simulink model "case2"  (R2024b)
settings: Solver=FixedStepAuto  StartTime=0  StopTime=1  FixedStep=1e-7  RelTol=1e-3
values from neighbouring files (symbols this model uses):
  SG_D_1_D = 0.01056    [IEEE9_case_parameters.m]    (also in case1_parameters.m; case2_parameters.m; case3_parameters.m; case4_parameters.m)
  SG_D_1_EnableSaturation = 0    [IEEE9_case_parameters.m]    (also in case1_parameters.m; case2_parameters.m; case3_parameters.m; case4_parameters.m)
  SG_D_1_f0 = 60    [IEEE9_case_parameters.m]    (also in case1_parameters.m; case2_parameters.m; case3_parameters.m; case4_parameters.m)
  SG_D_1_H = 7.5    [IEEE9_case_parameters.m]    (also in case1_parameters.m; case2_parameters.m; case3_parameters.m; case4_parameters.m)
  SG_D_1_K_A = 20    [IEEE9_case_parameters.m]    (also in case1_parameters.m; case2_parameters.m; case3_parameters.m; case4_parameters.m)
  SG_D_1_K_E = 1.000000e+1    (= 10)    [IEEE9_case_parameters.m]    (also in case1_parameters.m; case2_parameters.m; case3_parameters.m; case4_parameters.m)
  SG_D_1_K_F = 2.363    [IEEE9_case_parameters.m]    (also in case1_parameters.m; case2_parameters.m; case3_parameters.m; case4_parameters.m)
  SG_D_1_K_s = 0.5    [IEEE9_case_parameters.m]    (also in case1_parameters.m = 5; case2_parameters.m = 5; case3_parameters.m = 5; case4_parameters.m = 5)
  SG_D_1_R_a = 0.001088    [IEEE9_case_parameters.m]    (also in case1_parameters.m; case2_parameters.m; case3_parameters.m; case4_parameters.m)
  SG_D_1_S_A = 1    [IEEE9_case_parameters.m]    (also in case1_parameters.m; case2_parameters.m; case3_parameters.m; case4_parameters.m)
  SG_D_1_S_B = 0.103    [IEEE9_case_parameters.m]    (also in case1_parameters.m; case2_parameters.m; case3_parameters.m; case4_parameters.m)
  SG_D_1_S_N = 10.659857    [IEEE9_case_parameters.m]    (also in case1_parameters.m; case2_parameters.m; case3_parameters.m; case4_parameters.m)
  SG_D_1_SpeedPara = 200    [IEEE9_case_parameters.m]    (also in case1_parameters.m; case2_parameters.m; case3_parameters.m; case4_parameters.m)
  SG_D_1_T_0 = 0.720173    [IEEE9_case_parameters.m]    (also in case1_parameters.m = 0.755522; case2_parameters.m = 0.808931; case3_parameters.m = 0.869402; case4_parameters.m = 0.729316)
  SG_D_1_T_1 = 0.3    [IEEE9_case_parameters.m]    (also in case1_parameters.m; case2_parameters.m; case3_parameters.m; case4_parameters.m)
  SG_D_1_T_2 = 0.05    [IEEE9_case_parameters.m]    (also in case1_parameters.m; case2_parameters.m; case3_parameters.m; case4_parameters.m)
  SG_D_1_T_3 = 0.02    [IEEE9_case_parameters.m]    (also in case1_parameters.m; case2_parameters.m; case3_parameters.m; case4_parameters.m)
  SG_D_1_T_4 = 0.005    [IEEE9_case_parameters.m]    (also in case1_parameters.m; case2_parameters.m; case3_parameters.m; case4_parameters.m)
  SG_D_1_T_A = 0.02    [IEEE9_case_parameters.m]    (also in case1_parameters.m; case2_parameters.m; case3_parameters.m; case4_parameters.m)
  SG_D_1_T_dd = 8.000000e+0    (= 8)    [IEEE9_case_parameters.m]    (also in case1_parameters.m; case2_parameters.m; case3_parameters.m; case4_parameters.m)
  SG_D_1_T_ddd = 0.04    [IEEE9_case_parameters.m]    (also in case1_parameters.m; case2_parameters.m; case3_parameters.m; case4_parameters.m)
  SG_D_1_T_E = 0.314    [IEEE9_case_parameters.m]    (also in case1_parameters.m; case2_parameters.m; case3_parameters.m; case4_parameters.m)
  SG_D_1_T_F = 0.35    [IEEE9_case_parameters.m]    (also in case1_parameters.m; case2_parameters.m; case3_parameters.m; case4_parameters.m)
  SG_D_1_T_qd = 0.8    [IEEE9_case_parameters.m]    (also in case1_parameters.m; case2_parameters.m; case3_parameters.m; case4_parameters.m)
  SG_D_1_T_qdd = 0.02    [IEEE9_case_parameters.m]    (also in case1_parameters.m; case2_parameters.m; case3_parameters.m; case4_parameters.m)
  SG_D_1_T_speed = 0.1    [IEEE9_case_parameters.m]    (also in case1_parameters.m = 200; case2_parameters.m = 200; case3_parameters.m = 200; case4_parameters.m = 200)
  SG_D_1_T_w = 0.5    [IEEE9_case_parameters.m]    (also in case1_parameters.m; case2_parameters.m; case3_parameters.m; case4_parameters.m)
  SG_D_1_V_ref = 1.990276    [IEEE9_case_parameters.m]    (also in case1_parameters.m = 2.042296; case2_parameters.m = 2.051388; case3_parameters.m = 2.089584; case4_parameters.m = 2.01845)
  SG_D_1_w_ref = 376.991118    [IEEE9_case_parameters.m]    (also in case1_parameters.m; case2_parameters.m; case3_parameters.m; case4_parameters.m)
  SG_D_1_wb = 6.000000e+1    (= 60)    [IEEE9_case_parameters.m]    (also in case1_parameters.m; case2_parameters.m; case3_parameters.m; case4_parameters.m)
  SG_D_1_x_d = 1.9    [IEEE9_case_parameters.m]    (also in case1_parameters.m; case2_parameters.m; case3_parameters.m; case4_parameters.m)
  SG_D_1_x_dd = 0.302    [IEEE9_case_parameters.m]    (also in case1_parameters.m; case2_parameters.m; case3_parameters.m; case4_parameters.m)
  SG_D_1_x_ddd = 0.204    [IEEE9_case_parameters.m]    (also in case1_parameters.m; case2_parameters.m; case3_parameters.m; case4_parameters.m)
  SG_D_1_x_l = 0.05    [IEEE9_case_parameters.m]    (also in case1_parameters.m; case2_parameters.m; case3_parameters.m; case4_parameters.m)
  SG_D_1_x_q = 1.3    [IEEE9_case_parameters.m]    (also in case1_parameters.m; case2_parameters.m; case3_parameters.m; case4_parameters.m)
  SG_D_1_x_qd = 0.5    [IEEE9_case_parameters.m]    (also in case1_parameters.m; case2_parameters.m; case3_parameters.m; case4_parameters.m)
  SG_D_1_x_qdd = 0.3    [IEEE9_case_parameters.m]    (also in case1_parameters.m; case2_parameters.m; case3_parameters.m; case4_parameters.m)
  SG_D_2_D = 0.02    [IEEE9_case_parameters.m]    (also in case1_parameters.m; case2_parameters.m; case3_parameters.m; case4_parameters.m)
  SG_D_2_EnableSaturation = 0    [IEEE9_case_parameters.m]    (also in case1_parameters.m; case2_parameters.m; case3_parameters.m; case4_parameters.m)
  SG_D_2_f0 = 60    [IEEE9_case_parameters.m]    (also in case1_parameters.m; case2_parameters.m; case3_parameters.m; case4_parameters.m)
  SG_D_2_H = 8.000000e+0    (= 8)    [IEEE9_case_parameters.m]    (also in case1_parameters.m; case2_parameters.m; case3_parameters.m; case4_parameters.m)
  SG_D_2_K_A = 20    [IEEE9_case_parameters.m]    (also in case1_parameters.m; case2_parameters.m; case3_parameters.m; case4_parameters.m)
  SG_D_2_K_E = 1.000000e+1    (= 10)    [IEEE9_case_parameters.m]    (also in case1_parameters.m; case2_parameters.m; case3_parameters.m; case4_parameters.m)
  SG_D_2_K_F = 2.363    [IEEE9_case_parameters.m]    (also in case1_parameters.m; case2_parameters.m; case3_parameters.m; case4_parameters.m)
  SG_D_2_K_s = 0.5    [IEEE9_case_parameters.m]    (also in case1_parameters.m = 4; case2_parameters.m = 4; case3_parameters.m = 4; case4_parameters.m = 4)
  SG_D_2_R_a = 0.001088    [IEEE9_case_parameters.m]    (also in case1_parameters.m; case2_parameters.m; case3_parameters.m; case4_parameters.m)
  SG_D_2_S_A = 1    [IEEE9_case_parameters.m]    (also in case1_parameters.m; case2_parameters.m; case3_parameters.m; case4_parameters.m)
  SG_D_2_S_B = 0.103    [IEEE9_case_parameters.m]    (also in case1_parameters.m; case2_parameters.m; case3_parameters.m; case4_parameters.m)
  SG_D_2_S_N = 10.659857    [IEEE9_case_parameters.m]    (also in case1_parameters.m; case2_parameters.m; case3_parameters.m; case4_parameters.m)
  SG_D_2_SpeedPara = 200    [IEEE9_case_parameters.m]    (also in case1_parameters.m; case2_parameters.m; case3_parameters.m; case4_parameters.m)
  SG_D_2_T_0 = 1.632913    [IEEE9_case_parameters.m]    (also in case1_parameters.m = 1.632925; case2_parameters.m = 1.632915; case3_parameters.m = 1.632914; case4_parameters.m = 1.632927)
  SG_D_2_T_1 = 0.2    [IEEE9_case_parameters.m]    (also in case1_parameters.m; case2_parameters.m; case3_parameters.m; case4_parameters.m)
  SG_D_2_T_2 = 0.05    [IEEE9_case_parameters.m]    (also in case1_parameters.m; case2_parameters.m; case3_parameters.m; case4_parameters.m)
  SG_D_2_T_3 = 0.02    [IEEE9_case_parameters.m]    (also in case1_parameters.m; case2_parameters.m; case3_parameters.m; case4_parameters.m)
  SG_D_2_T_4 = 0.005    [IEEE9_case_parameters.m]    (also in case1_parameters.m; case2_parameters.m; case3_parameters.m; case4_parameters.m)
  SG_D_2_T_A = 0.02    [IEEE9_case_parameters.m]    (also in case1_parameters.m; case2_parameters.m; case3_parameters.m; case4_parameters.m)
  SG_D_2_T_dd = 7.9    [IEEE9_case_parameters.m]    (also in case1_parameters.m; case2_parameters.m; case3_parameters.m; case4_parameters.m)
  SG_D_2_T_ddd = 0.04    [IEEE9_case_parameters.m]    (also in case1_parameters.m; case2_parameters.m; case3_parameters.m; case4_parameters.m)
  SG_D_2_T_E = 0.314    [IEEE9_case_parameters.m]    (also in case1_parameters.m; case2_parameters.m; case3_parameters.m; case4_parameters.m)
  SG_D_2_T_F = 0.35    [IEEE9_case_parameters.m]    (also in case1_parameters.m; case2_parameters.m; case3_parameters.m; case4_parameters.m)
  SG_D_2_T_qd = 0.8    [IEEE9_case_parameters.m]    (also in case1_parameters.m; case2_parameters.m; case3_parameters.m; case4_parameters.m)
  SG_D_2_T_qdd = 0.015    [IEEE9_case_parameters.m]    (also in case1_parameters.m; case2_parameters.m; case3_parameters.m; case4_parameters.m)
  SG_D_2_T_speed = 0.1    [IEEE9_case_parameters.m]    (also in case1_parameters.m = 150; case2_parameters.m = 150; case3_parameters.m = 150; case4_parameters.m = 150)
  SG_D_2_T_w = 0.35    [IEEE9_case_parameters.m]    (also in case1_parameters.m; case2_parameters.m; case3_parameters.m; case4_parameters.m)
  SG_D_2_V_ref = 2.58547    [IEEE9_case_parameters.m]    (also in case1_parameters.m = 2.597896; case2_parameters.m = 2.587136; case3_parameters.m = 2.586042; case4_parameters.m = 2.599679)
  SG_D_2_w_ref = 376.991118    [IEEE9_case_parameters.m]    (also in case1_parameters.m; case2_parameters.m; case3_parameters.m; case4_parameters.m)
  SG_D_2_wb = 6.000000e+1    (= 60)    [IEEE9_case_parameters.m]    (also in case1_parameters.m; case2_parameters.m; case3_parameters.m; case4_parameters.m)
  SG_D_2_x_d = 1.8    [IEEE9_case_parameters.m]    (also in case1_parameters.m; case2_parameters.m; case3_parameters.m; case4_parameters.m)
  SG_D_2_x_dd = 0.302    [IEEE9_case_parameters.m]    (also in case1_parameters.m; case2_parameters.m; case3_parameters.m; case4_parameters.m)
  SG_D_2_x_ddd = 0.204    [IEEE9_case_parameters.m]    (also in case1_parameters.m; case2_parameters.m; case3_parameters.m; case4_parameters.m)
  SG_D_2_x_l = 0.05    [IEEE9_case_parameters.m]    (also in case1_parameters.m; case2_parameters.m; case3_parameters.m; case4_parameters.m)
  SG_D_2_x_q = 1.25    [IEEE9_case_parameters.m]    (also in case1_parameters.m; case2_parameters.m; case3_parameters.m; case4_parameters.m)
  SG_D_2_x_qd = 0.5    [IEEE9_case_parameters.m]    (also in case1_parameters.m; case2_parameters.m; case3_parameters.m; case4_parameters.m)
  SG_D_2_x_qdd = 0.3    [IEEE9_case_parameters.m]    (also in case1_parameters.m; case2_parameters.m; case3_parameters.m; case4_parameters.m)
  SG_D_3_D = 0.02    [IEEE9_case_parameters.m]    (also in case1_parameters.m; case2_parameters.m; case3_parameters.m; case4_parameters.m)
  SG_D_3_EnableSaturation = 0    [IEEE9_case_parameters.m]    (also in case1_parameters.m; case2_parameters.m; case3_parameters.m; case4_parameters.m)
  SG_D_3_f0 = 60    [IEEE9_case_parameters.m]    (also in case1_parameters.m; case2_parameters.m; case3_parameters.m; case4_parameters.m)
  SG_D_3_H = 7.7    [IEEE9_case_parameters.m]    (also in case1_parameters.m; case2_parameters.m; case3_parameters.m; case4_parameters.m)
  SG_D_3_K_A = 20    [IEEE9_case_parameters.m]    (also in case1_parameters.m; case2_parameters.m; case3_parameters.m; case4_parameters.m)
  SG_D_3_K_E = 1.000000e+1    (= 10)    [IEEE9_case_parameters.m]    (also in case1_parameters.m; case2_parameters.m; case3_parameters.m; case4_parameters.m)
  SG_D_3_K_F = 2.363    [IEEE9_case_parameters.m]    (also in case1_parameters.m; case2_parameters.m; case3_parameters.m; case4_parameters.m)
  SG_D_3_K_s = 0.2    [IEEE9_case_parameters.m]    (also in case1_parameters.m = 2; case2_parameters.m = 2; case3_parameters.m = 2; case4_parameters.m = 2)
  SG_D_3_R_a = 0.001088    [IEEE9_case_parameters.m]    (also in case1_parameters.m; case2_parameters.m; case3_parameters.m; case4_parameters.m)
  SG_D_3_S_A = 1    [IEEE9_case_parameters.m]    (also in case1_parameters.m; case2_parameters.m; case3_parameters.m; case4_parameters.m)
  SG_D_3_S_B = 0.103    [IEEE9_case_parameters.m]    (also in case1_parameters.m; case2_parameters.m; case3_parameters.m; case4_parameters.m)
  SG_D_3_S_N = 10.659857    [IEEE9_case_parameters.m]    (also in case1_parameters.m; case2_parameters.m; case3_parameters.m; case4_parameters.m)
  SG_D_3_SpeedPara = 200    [IEEE9_case_parameters.m]    (also in case1_parameters.m; case2_parameters.m; case3_parameters.m; case4_parameters.m)
  SG_D_3_T_0 = 0.850788    [IEEE9_case_parameters.m]    (also in case1_parameters.m = 0.850786; case2_parameters.m = 0.850787; case3_parameters.m; case4_parameters.m = 0.850786)
  SG_D_3_T_1 = 0.2    [IEEE9_case_parameters.m]    (also in case1_parameters.m; case2_parameters.m; case3_parameters.m; case4_parameters.m)
  SG_D_3_T_2 = 0.05    [IEEE9_case_parameters.m]    (also in case1_parameters.m; case2_parameters.m; case3_parameters.m; case4_parameters.m)
  SG_D_3_T_3 = 0.02    [IEEE9_case_parameters.m]    (also in case1_parameters.m; case2_parameters.m; case3_parameters.m; case4_parameters.m)
  SG_D_3_T_4 = 0.005    [IEEE9_case_parameters.m]    (also in case1_parameters.m; case2_parameters.m; case3_parameters.m; case4_parameters.m)
  SG_D_3_T_A = 0.02    [IEEE9_case_parameters.m]    (also in case1_parameters.m; case2_parameters.m; case3_parameters.m; case4_parameters.m)
  SG_D_3_T_dd = 8.1    [IEEE9_case_parameters.m]    (also in case1_parameters.m; case2_parameters.m; case3_parameters.m; case4_parameters.m)
  SG_D_3_T_ddd = 0.04    [IEEE9_case_parameters.m]    (also in case1_parameters.m; case2_parameters.m; case3_parameters.m; case4_parameters.m)
  SG_D_3_T_E = 0.314    [IEEE9_case_parameters.m]    (also in case1_parameters.m; case2_parameters.m; case3_parameters.m; case4_parameters.m)
  SG_D_3_T_F = 0.35    [IEEE9_case_parameters.m]    (also in case1_parameters.m; case2_parameters.m; case3_parameters.m; case4_parameters.m)
  SG_D_3_T_qd = 0.8    [IEEE9_case_parameters.m]    (also in case1_parameters.m; case2_parameters.m; case3_parameters.m; case4_parameters.m)
  SG_D_3_T_qdd = 0.015    [IEEE9_case_parameters.m]    (also in case1_parameters.m; case2_parameters.m; case3_parameters.m; case4_parameters.m)
  SG_D_3_T_speed = 0.1    [IEEE9_case_parameters.m]    (also in case1_parameters.m = 180; case2_parameters.m = 180; case3_parameters.m = 180; case4_parameters.m = 180)
  SG_D_3_T_w = 0.4    [IEEE9_case_parameters.m]    (also in case1_parameters.m; case2_parameters.m; case3_parameters.m; case4_parameters.m)
  SG_D_3_V_ref = 1.892727    [IEEE9_case_parameters.m]    (also in case1_parameters.m = 1.906439; case2_parameters.m = 1.895535; case3_parameters.m = 1.892105; case4_parameters.m = 1.906598)
  SG_D_3_w_ref = 376.991118    [IEEE9_case_parameters.m]    (also in case1_parameters.m; case2_parameters.m; case3_parameters.m; case4_parameters.m)
  SG_D_3_wb = 6.000000e+1    (= 60)    [IEEE9_case_parameters.m]    (also in case1_parameters.m; case2_parameters.m; case3_parameters.m; case4_parameters.m)
  SG_D_3_x_d = 1.85    [IEEE9_case_parameters.m]    (also in case1_parameters.m; case2_parameters.m; case3_parameters.m; case4_parameters.m)
  SG_D_3_x_dd = 0.302    [IEEE9_case_parameters.m]    (also in case1_parameters.m; case2_parameters.m; case3_parameters.m; case4_parameters.m)
  SG_D_3_x_ddd = 0.204    [IEEE9_case_parameters.m]    (also in case1_parameters.m; case2_parameters.m; case3_parameters.m; case4_parameters.m)
  SG_D_3_x_l = 0.05    [IEEE9_case_parameters.m]    (also in case1_parameters.m; case2_parameters.m; case3_parameters.m; case4_parameters.m)
  SG_D_3_x_q = 1.2    [IEEE9_case_parameters.m]    (also in case1_parameters.m; case2_parameters.m; case3_parameters.m; case4_parameters.m)
  SG_D_3_x_qd = 0.5    [IEEE9_case_parameters.m]    (also in case1_parameters.m; case2_parameters.m; case3_parameters.m; case4_parameters.m)
  SG_D_3_x_qdd = 0.3    [IEEE9_case_parameters.m]    (also in case1_parameters.m; case2_parameters.m; case3_parameters.m; case4_parameters.m)
(part 9 of 12)

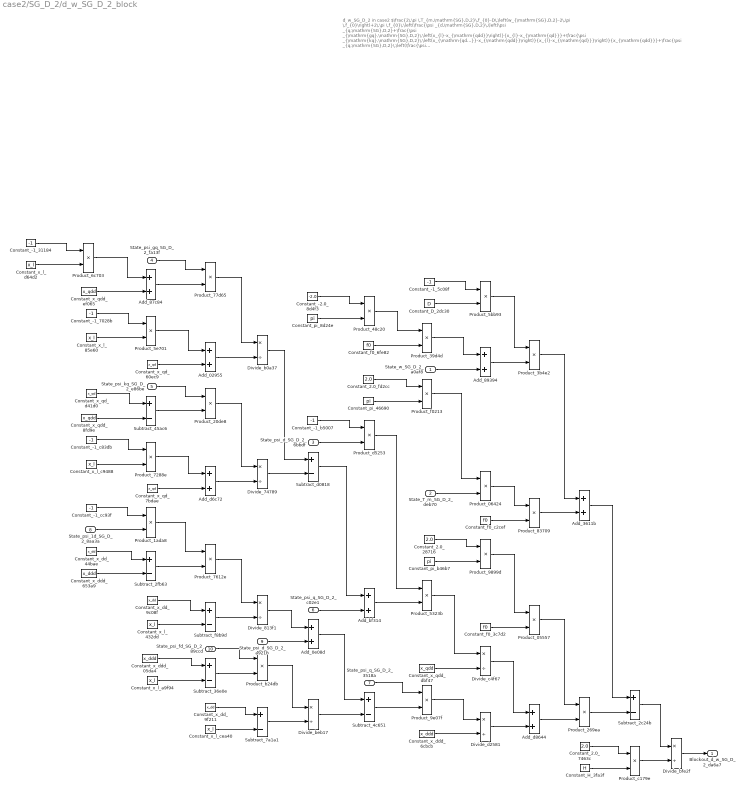
== system case2/SG_D_2/d_w_SG_D_2_block ==
  note: d_w_SG_D_2 in case2
      | $\frac{2\,\pi \,T_{m,\mathrm{SG},D,2}\,f_{0}-D\,\left(w_{\mathrm{SG},D,2}-2\,\pi \,f_{0}\right)+2\,\pi \,f_{0}\,\left(\frac{\psi _{d,\mathrm{SG},D,2}\,\left(\psi _{q,\mathrm{SG},D,2}+\frac{\psi _{\mathrm{gq},\mathrm{SG},D,2}\,\left(x_{l}-x_{\mathrm{qdd}}\right)}{x_{l}-x_{\mathrm{qd}}}+\frac{\psi _{\mathrm{kq},\mathrm{SG},D,2}\,\left(x_{\mathrm{qd}}-x_{\mathrm{qdd}}\right)}{x_{l}-x_{\mathrm{qd}}}\right)}{x_{\mathrm{qdd}}}+\frac{\psi _{q,\mathrm{SG},D,2}\,\left(\frac{\psi _{\mathrm{1d},\mathrm{SG},D,2}\,\left(x_{\mathrm{dd}}-x_{\mathrm{ddd}}\right)}{x_{\mathrm{dd}}-x_{l}}-\psi _{d,\mathrm{SG},D,2}+\frac{\psi _{\mathrm{fd},\mathrm{SG},D,2}\,\left(x_{\mathrm{ddd}}-x_{l}\right)}{x_{\mathrm{dd}}-x_{l}}\right)}{x_{\mathrm{ddd}}}\right)}{2\,H}$
      | Automatically generated on 2025-10-31 18:54:39 .
  State_w_SG_D_2_a0af8 : Inport
  State_T_m_SG_D_2_deb70 : Inport  Port=2
  State_psi_d_SG_D_2_6bbdf : Inport  Port=3
  State_psi_gq_SG_D_2_fa13f : Inport  Port=4
  State_psi_kq_SG_D_2_e86be : Inport  Port=5
  State_psi_q_SG_D_2_c02e1 : Inport  Port=6
  State_psi_q_SG_D_2_3518a : Inport  Port=7
  State_psi_1d_SG_D_2_8aa3a : Inport  Port=8
  State_psi_d_SG_D_2_a921b : Inport  Port=9
  State_psi_fd_SG_D_2_89ccd : Inport  Port=10
  Add_02955 : Sum
  Add_0e08d : Sum
  Add_3611b : Sum
  Add_87c84 : Sum
  Add_89394 : Sum
  Add_bf314 : Sum
  Add_d6c72 : Sum
  Add_d8644 : Sum
  Constant_-1_31184 : Constant  Value=-1
  Constant_-1_5c08f : Constant  Value=-1
  Constant_-1_7028b : Constant  Value=-1
  Constant_-1_b5007 : Constant  Value=-1
  Constant_-1_c83db : Constant  Value=-1
  Constant_-1_cc93f : Constant  Value=-1
  Constant_-2.0_8d4f3 : Constant  Value=-2.0
  Constant_2.0_28716 : Constant  Value=2.0
  Constant_2.0_7463c : Constant  Value=2.0
  Constant_2.0_fd2cc : Constant  Value=2.0
  Constant_D_2dc30 : Constant  Value=D
  Constant_H_3fa3f : Constant  Value=H
  Constant_f0_3c7d2 : Constant  Value=f0
  Constant_f0_6fe82 : Constant  Value=f0
  Constant_f0_c2cef : Constant  Value=f0
  Constant_pi_46690 : Constant  Value=pi
  Constant_pi_8d24e : Constant  Value=pi
  Constant_pi_b46b7 : Constant  Value=pi
  Constant_x_dd_44bae : Constant  Value=x_dd
  Constant_x_dd_9c08f : Constant  Value=x_dd
  Constant_x_dd_9f211 : Constant  Value=x_dd
  Constant_x_ddd_05da4 : Constant  Value=x_ddd
  Constant_x_ddd_653a9 : Constant  Value=x_ddd
  Constant_x_ddd_6cbcb : Constant  Value=x_ddd
  Constant_x_l_432dd : Constant  Value=x_l
  Constant_x_l_85e60 : Constant  Value=x_l
  Constant_x_l_a9f94 : Constant  Value=x_l
  Constant_x_l_c9488 : Constant  Value=x_l
  Constant_x_l_cea40 : Constant  Value=x_l
  Constant_x_l_d64d2 : Constant  Value=x_l
  Constant_x_qd_60ec9 : Constant  Value=x_qd
  Constant_x_qd_7bdae : Constant  Value=x_qd
  Constant_x_qd_d41d0 : Constant  Value=x_qd
  Constant_x_qdd_8fd9e : Constant  Value=x_qdd
  Constant_x_qdd_dbf47 : Constant  Value=x_qdd
  Constant_x_qdd_ef065 : Constant  Value=x_qdd
  Divide_74789 : Product  Inputs=*/
  Divide_813f1 : Product  Inputs=*/
  Divide_b0a37 : Product  Inputs=*/
  Divide_beb17 : Product  Inputs=*/
  Divide_bfe2f : Product  Inputs=*/
  Divide_c4f67 : Product  Inputs=*/
  Divide_d2581 : Product  Inputs=*/
  Product_05557 : Product
  Product_06424 : Product
  Product_1ada8 : Product
  Product_20de8 : Product
  Product_269ea : Product
  Product_39d4d : Product
  Product_3b4e2 : Product
  Product_48c20 : Product
  Product_5323b : Product
  Product_5bb93 : Product
  Product_5e701 : Product
  Product_6c703 : Product
  Product_7288e : Product
  Product_7612e : Product
  Product_77d65 : Product
  Product_83709 : Product
  Product_9899d : Product
  Product_9e07f : Product
  Product_b24db : Product
  Product_c179e : Product
  Product_d5253 : Product
  Product_f0213 : Product
  Subtract_2c24b : Sum  Inputs=+-
  Subtract_2fb63 : Sum  Inputs=+-
  Subtract_36e0e : Sum  Inputs=+-
  Subtract_45ac6 : Sum  Inputs=+-
  Subtract_4c651 : Sum  Inputs=+-
  Subtract_7a1a1 : Sum  Inputs=+-
  Subtract_d0818 : Sum  Inputs=+-
  Subtract_f8b9d : Sum  Inputs=+-
  Blockout_d_w_SG_D_2_da6a7 : Outport
  wires:
  Constant_x_qd_d41d0/1 -> Subtract_45ac6/1
  Constant_-1_c83db/1 -> Product_7288e/1
  Constant_-1_31184/1 -> Product_6c703/1
  Constant_x_qdd_8fd9e/1 -> Subtract_45ac6/2
  Subtract_7a1a1/1 -> Divide_beb17/2
  Constant_x_l_c9488/1 -> Product_7288e/2
  Constant_x_l_d64d2/1 -> Product_6c703/2
  Product_7288e/1 -> Add_d6c72/1
  Product_6c703/1 -> Add_87c84/1
  Constant_x_l_432dd/1 -> Subtract_f8b9d/2
  Constant_x_l_85e60/1 -> Product_5e701/2
  Constant_x_ddd_6cbcb/1 -> Divide_d2581/2
  Subtract_36e0e/1 -> Product_b24db/2
  Constant_x_qd_7bdae/1 -> Add_d6c72/2
  Constant_x_qdd_ef065/1 -> Add_87c84/2
  Constant_-1_7028b/1 -> Product_5e701/1
  State_psi_d_SG_D_2_6bbdf/1 -> Product_d5253/2
  Constant_-1_cc93f/1 -> Product_1ada8/1
  State_w_SG_D_2_a0af8/1 -> Add_89394/2
  Product_5e701/1 -> Add_02955/1
  State_psi_1d_SG_D_2_8aa3a/1 -> Product_1ada8/2
  Constant_x_dd_44bae/1 -> Subtract_2fb63/1
  Divide_b0a37/1 -> Subtract_d0818/1
  Subtract_45ac6/1 -> Product_20de8/2
  Constant_x_ddd_653a9/1 -> Subtract_2fb63/2
  State_psi_gq_SG_D_2_fa13f/1 -> Product_77d65/1
  Add_d6c72/1 -> Divide_74789/2
  State_psi_d_SG_D_2_a921b/1 -> Add_0e08d/2
  Add_87c84/1 -> Product_77d65/2
  Constant_x_qd_60ec9/1 -> Add_02955/2
  State_psi_kq_SG_D_2_e86be/1 -> Product_20de8/1
  Product_1ada8/1 -> Product_7612e/1
  Subtract_2fb63/1 -> Product_7612e/2
  Constant_pi_46690/1 -> Product_f0213/2
  Constant_x_dd_9c08f/1 -> Subtract_f8b9d/1
  Constant_x_ddd_05da4/1 -> Subtract_36e0e/1
  Constant_x_l_a9f94/1 -> Subtract_36e0e/2
  Product_77d65/1 -> Divide_b0a37/1
  Add_02955/1 -> Divide_b0a37/2
  Add_bf314/1 -> Product_5323b/2
  Product_20de8/1 -> Divide_74789/1
  Constant_pi_8d24e/1 -> Product_48c20/2
  Product_7612e/1 -> Divide_813f1/1
  Subtract_f8b9d/1 -> Divide_813f1/2
  State_psi_fd_SG_D_2_89ccd/1 -> Product_b24db/1
  Divide_813f1/1 -> Add_0e08d/1
  Constant_x_dd_9f211/1 -> Subtract_7a1a1/1
  Constant_x_l_cea40/1 -> Subtract_7a1a1/2
  Divide_74789/1 -> Subtract_d0818/2
  Product_b24db/1 -> Divide_beb17/1
  Constant_-1_b5007/1 -> Product_d5253/1
  Constant_-2.0_8d4f3/1 -> Product_48c20/1
  Subtract_d0818/1 -> Add_bf314/1
  Subtract_4c651/1 -> Product_9e07f/2
  State_psi_q_SG_D_2_c02e1/1 -> Add_bf314/2
  Constant_D_2dc30/1 -> Product_5bb93/2
  Add_0e08d/1 -> Subtract_4c651/1
  Divide_beb17/1 -> Subtract_4c651/2
  Product_48c20/1 -> Product_39d4d/1
  Constant_f0_6fe82/1 -> Product_39d4d/2
  Constant_2.0_fd2cc/1 -> Product_f0213/1
  Product_d5253/1 -> Product_5323b/1
  State_psi_q_SG_D_2_3518a/1 -> Product_9e07f/1
  Constant_-1_5c08f/1 -> Product_5bb93/1
  Product_39d4d/1 -> Add_89394/1
  Product_f0213/1 -> Product_06424/1
  State_T_m_SG_D_2_deb70/1 -> Product_06424/2
  Constant_2.0_28716/1 -> Product_9899d/1
  Constant_pi_b46b7/1 -> Product_9899d/2
  Product_5323b/1 -> Divide_c4f67/1
  Constant_x_qdd_dbf47/1 -> Divide_c4f67/2
  Product_9e07f/1 -> Divide_d2581/1
  Product_5bb93/1 -> Product_3b4e2/1
  Add_89394/1 -> Product_3b4e2/2
  Product_06424/1 -> Product_83709/1
  Constant_f0_c2cef/1 -> Product_83709/2
  Product_9899d/1 -> Product_05557/1
  Constant_f0_3c7d2/1 -> Product_05557/2
  Divide_c4f67/1 -> Add_d8644/1
  Divide_d2581/1 -> Add_d8644/2
  Product_3b4e2/1 -> Add_3611b/1
  Product_83709/1 -> Add_3611b/2
  Product_05557/1 -> Product_269ea/1
  Add_d8644/1 -> Product_269ea/2
  Add_3611b/1 -> Subtract_2c24b/1
  Product_269ea/1 -> Subtract_2c24b/2
  Constant_2.0_7463c/1 -> Product_c179e/1
  Constant_H_3fa3f/1 -> Product_c179e/2
  Subtract_2c24b/1 -> Divide_bfe2f/1
  Product_c179e/1 -> Divide_bfe2f/2
  Divide_bfe2f/1 -> Blockout_d_w_SG_D_2_da6a7/1

== system case2/SG_D_2/i_d_SG_D_2_block ==
  note: i_d_SG_D_2 in case2
      | $\frac{\sin\left(\theta _{\mathrm{SG},D,2}\right)\,\left(\frac{\psi _{\mathrm{1d},\mathrm{SG},D,2}\,\left(x_{\mathrm{dd}}-x_{\mathrm{ddd}}\right)}{x_{\mathrm{dd}}-x_{l}}-\psi _{d,\mathrm{SG},D,2}+\frac{\psi _{\mathrm{fd},\mathrm{SG},D,2}\,\left(x_{\mathrm{ddd}}-x_{l}\right)}{x_{\mathrm{dd}}-x_{l}}\right)}{x_{\mathrm{ddd}}}-\frac{\cos\left(\theta _{\mathrm{SG},D,2}\right)\,\left(\psi _{q,\mathrm{SG},D,2}+\frac{\psi _{\mathrm{gq},\mathrm{SG},D,2}\,\left(x_{l}-x_{\mathrm{qdd}}\right)}{x_{l}-x_{\mathrm{qd}}}+\frac{\psi _{\mathrm{kq},\mathrm{SG},D,2}\,\left(x_{\mathrm{qd}}-x_{\mathrm{qdd}}\right)}{x_{l}-x_{\mathrm{qd}}}\right)}{x_{\mathrm{qdd}}}$
      | Automatically generated on 2025-10-31 18:55:03 .
  State_psi_gq_SG_D_2_419a5 : Inport
  State_psi_kq_SG_D_2_2885e : Inport  Port=2
  State_psi_q_SG_D_2_74918 : Inport  Port=3
  State_theta_SG_D_2_67c6e : Inport  Port=4
  State_psi_1d_SG_D_2_37338 : Inport  Port=5
  State_psi_d_SG_D_2_8c17d : Inport  Port=6
  State_psi_fd_SG_D_2_463f2 : Inport  Port=7
  State_theta_SG_D_2_e4d3c : Inport  Port=8
  Add_0dc8a : Sum
  Add_1a230 : Sum
  Add_93dd7 : Sum
  Add_9db99 : Sum
  Add_ff8c8 : Sum
  Constant_-1_3e56d : Constant  Value=-1
  Constant_-1_4eb79 : Constant  Value=-1
  Constant_-1_7a55c : Constant  Value=-1
  Constant_-1_9666d : Constant  Value=-1
  Constant_-1_dbe66 : Constant  Value=-1
  Constant_x_dd_bc375 : Constant  Value=x_dd
  Constant_x_dd_e4e31 : Constant  Value=x_dd
  Constant_x_dd_fc25d : Constant  Value=x_dd
  Constant_x_ddd_2e550 : Constant  Value=x_ddd
  Constant_x_ddd_ddfca : Constant  Value=x_ddd
  Constant_x_ddd_e08ae : Constant  Value=x_ddd
  Constant_x_l_18470 : Constant  Value=x_l
  Constant_x_l_71f42 : Constant  Value=x_l
  Constant_x_l_90b74 : Constant  Value=x_l
  Constant_x_l_956e8 : Constant  Value=x_l
  Constant_x_l_d5539 : Constant  Value=x_l
  Constant_x_l_f6f09 : Constant  Value=x_l
  Constant_x_qd_12c30 : Constant  Value=x_qd
  Constant_x_qd_96535 : Constant  Value=x_qd
  Constant_x_qd_d44b4 : Constant  Value=x_qd
  Constant_x_qdd_396df : Constant  Value=x_qdd
  Constant_x_qdd_a7674 : Constant  Value=x_qdd
  Constant_x_qdd_b7322 : Constant  Value=x_qdd
  Divide_426be : Product  Inputs=*/
  Divide_4bf7b : Product  Inputs=*/
  Divide_91a17 : Product  Inputs=*/
  Divide_a8dcd : Product  Inputs=*/
  Divide_f887f : Product  Inputs=*/
  Divide_fa9e8 : Product  Inputs=*/
  MathFunc_cos_09f11 : Trigonometry  Operator=cos
  MathFunc_sin_97974 : Trigonometry
  Product_1dd6b : Product
  Product_506ec : Product
  Product_6aa1c : Product
  Product_735e6 : Product
  Product_848ce : Product
  Product_ac690 : Product
  Product_bec85 : Product
  Product_dbe96 : Product
  Product_f820f : Product
  Product_fdbcd : Product
  Product_fecd3 : Product
  Subtract_238ed : Sum  Inputs=+-
  Subtract_26dad : Sum  Inputs=+-
  Subtract_3b1fc : Sum  Inputs=+-
  Subtract_6a710 : Sum  Inputs=+-
  Subtract_6a8c2 : Sum  Inputs=+-
  Subtract_8f6e9 : Sum  Inputs=+-
  Subtract_933eb : Sum  Inputs=+-
  Subtract_f60f0 : Sum  Inputs=+-
  Blockout_i_d_SG_D_2_4df8b : Outport
  wires:
  Constant_x_ddd_e08ae/1 -> Subtract_f60f0/1
  Constant_x_qd_d44b4/1 -> Subtract_26dad/1
  Constant_-1_9666d/1 -> Product_6aa1c/1
  Constant_-1_3e56d/1 -> Product_f820f/1
  Subtract_933eb/1 -> Blockout_i_d_SG_D_2_4df8b/1
  Constant_x_qdd_a7674/1 -> Subtract_26dad/2
  Constant_x_l_f6f09/1 -> Product_6aa1c/2
  Constant_x_l_956e8/1 -> Product_f820f/2
  Product_6aa1c/1 -> Add_93dd7/1
  Product_f820f/1 -> Add_9db99/1
  Constant_x_l_71f42/1 -> Product_fecd3/2
  Constant_x_qd_96535/1 -> Add_93dd7/2
  Constant_x_qdd_b7322/1 -> Add_9db99/2
  Constant_x_qdd_396df/1 -> Divide_426be/2
  MathFunc_cos_09f11/1 -> Product_bec85/2
  Constant_-1_dbe66/1 -> Product_fecd3/1
  State_psi_gq_SG_D_2_419a5/1 -> Product_1dd6b/1
  Subtract_f60f0/1 -> Product_506ec/2
  Product_848ce/1 -> Product_ac690/1
  Add_93dd7/1 -> Divide_4bf7b/2
  Add_9db99/1 -> Product_1dd6b/2
  Product_506ec/1 -> Divide_fa9e8/1
  Product_fecd3/1 -> Add_1a230/1
  Constant_x_qd_12c30/1 -> Add_1a230/2
  State_theta_SG_D_2_e4d3c/1 -> MathFunc_sin_97974/1
  State_psi_kq_SG_D_2_2885e/1 -> Product_735e6/1
  Add_0dc8a/1 -> Subtract_3b1fc/1
  Subtract_26dad/1 -> Product_735e6/2
  Product_1dd6b/1 -> Divide_f887f/1
  Constant_-1_4eb79/1 -> Product_848ce/1
  State_psi_1d_SG_D_2_37338/1 -> Product_848ce/2
  State_psi_fd_SG_D_2_463f2/1 -> Product_506ec/1
  Constant_x_dd_bc375/1 -> Subtract_238ed/1
  Product_ac690/1 -> Divide_91a17/1
  Constant_x_ddd_2e550/1 -> Subtract_238ed/2
  Divide_fa9e8/1 -> Subtract_3b1fc/2
  Add_1a230/1 -> Divide_f887f/2
  Product_dbe96/1 -> Divide_a8dcd/1
  Product_735e6/1 -> Divide_4bf7b/1
  Constant_-1_7a55c/1 -> Product_fdbcd/1
  Subtract_6a8c2/1 -> Divide_fa9e8/2
  Subtract_238ed/1 -> Product_ac690/2
  Constant_x_dd_fc25d/1 -> Subtract_8f6e9/1
  Subtract_3b1fc/1 -> Product_dbe96/1
  Constant_x_l_d5539/1 -> Subtract_8f6e9/2
  Constant_x_l_18470/1 -> Subtract_f60f0/2
  Divide_f887f/1 -> Subtract_6a710/1
  Divide_a8dcd/1 -> Subtract_933eb/2
  Divide_4bf7b/1 -> Subtract_6a710/2
  Subtract_8f6e9/1 -> Divide_91a17/2
  Constant_x_dd_e4e31/1 -> Subtract_6a8c2/1
  Divide_426be/1 -> Subtract_933eb/1
  Constant_x_l_90b74/1 -> Subtract_6a8c2/2
  Subtract_6a710/1 -> Add_ff8c8/1
  State_psi_q_SG_D_2_74918/1 -> Add_ff8c8/2
  Constant_x_ddd_ddfca/1 -> Divide_a8dcd/2
  MathFunc_sin_97974/1 -> Product_dbe96/2
  Divide_91a17/1 -> Add_0dc8a/1
  State_psi_d_SG_D_2_8c17d/1 -> Add_0dc8a/2
  Add_ff8c8/1 -> Product_fdbcd/2
  State_theta_SG_D_2_67c6e/1 -> MathFunc_cos_09f11/1
  Product_fdbcd/1 -> Product_bec85/1
  Product_bec85/1 -> Divide_426be/1

== system case2/SG_D_2/i_q_SG_D_2_block ==
  note: i_q_SG_D_2 in case2
      | $-\frac{\sin\left(\theta _{\mathrm{SG},D,2}\right)\,\left(\psi _{q,\mathrm{SG},D,2}+\frac{\psi _{\mathrm{gq},\mathrm{SG},D,2}\,\left(x_{l}-x_{\mathrm{qdd}}\right)}{x_{l}-x_{\mathrm{qd}}}+\frac{\psi _{\mathrm{kq},\mathrm{SG},D,2}\,\left(x_{\mathrm{qd}}-x_{\mathrm{qdd}}\right)}{x_{l}-x_{\mathrm{qd}}}\right)}{x_{\mathrm{qdd}}}-\frac{\cos\left(\theta _{\mathrm{SG},D,2}\right)\,\left(\frac{\psi _{\mathrm{1d},\mathrm{SG},D,2}\,\left(x_{\mathrm{dd}}-x_{\mathrm{ddd}}\right)}{x_{\mathrm{dd}}-x_{l}}-\psi _{d,\mathrm{SG},D,2}+\frac{\psi _{\mathrm{fd},\mathrm{SG},D,2}\,\left(x_{\mathrm{ddd}}-x_{l}\right)}{x_{\mathrm{dd}}-x_{l}}\right)}{x_{\mathrm{ddd}}}$
      | Automatically generated on 2025-10-31 18:55:07 .
  State_psi_gq_SG_D_2_62065 : Inport
  State_psi_kq_SG_D_2_46994 : Inport  Port=2
  State_psi_q_SG_D_2_d1f7c : Inport  Port=3
  State_theta_SG_D_2_14f06 : Inport  Port=4
  State_psi_1d_SG_D_2_3e03a : Inport  Port=5
  State_psi_d_SG_D_2_1a46c : Inport  Port=6
  State_psi_fd_SG_D_2_212cc : Inport  Port=7
  State_theta_SG_D_2_6d11f : Inport  Port=8
  Add_56e92 : Sum
  Add_61347 : Sum
  Add_b2275 : Sum
  Add_d2493 : Sum
  Add_da261 : Sum
  Add_dbe16 : Sum
  Constant_-1_31208 : Constant  Value=-1
  Constant_-1_31adc : Constant  Value=-1
  Constant_-1_d6b5e : Constant  Value=-1
  Constant_-1_d8871 : Constant  Value=-1
  Constant_-1_df0dd : Constant  Value=-1
  Constant_x_dd_3bc88 : Constant  Value=x_dd
  Constant_x_dd_9c14e : Constant  Value=x_dd
  Constant_x_dd_b221d : Constant  Value=x_dd
  Constant_x_ddd_677e6 : Constant  Value=x_ddd
  Constant_x_ddd_709cf : Constant  Value=x_ddd
  Constant_x_ddd_e9928 : Constant  Value=x_ddd
  Constant_x_l_0134d : Constant  Value=x_l
  Constant_x_l_3454d : Constant  Value=x_l
  Constant_x_l_699e0 : Constant  Value=x_l
  Constant_x_l_c5593 : Constant  Value=x_l
  Constant_x_l_f5f84 : Constant  Value=x_l
  Constant_x_l_fd7b2 : Constant  Value=x_l
  Constant_x_qd_9ab83 : Constant  Value=x_qd
  Constant_x_qd_a957b : Constant  Value=x_qd
  Constant_x_qd_fd3a7 : Constant  Value=x_qd
  Constant_x_qdd_75035 : Constant  Value=x_qdd
  Constant_x_qdd_c2e2f : Constant  Value=x_qdd
  Constant_x_qdd_fb9fa : Constant  Value=x_qdd
  Divide_36c98 : Product  Inputs=*/
  Divide_4487d : Product  Inputs=*/
  Divide_62534 : Product  Inputs=*/
  Divide_70422 : Product  Inputs=*/
  Divide_d545d : Product  Inputs=*/
  Divide_e9059 : Product  Inputs=*/
  MathFunc_cos_56f7a : Trigonometry  Operator=cos
  MathFunc_sin_69210 : Trigonometry
  Product_46ec5 : Product
  Product_5e931 : Product
  Product_6790a : Product
  Product_6dc77 : Product
  Product_7ddb9 : Product
  Product_89ab6 : Product
  Product_8d08d : Product
  Product_b81bd : Product
  Product_beae7 : Product
  Product_e4b88 : Product
  Product_ee3ef : Product
  Subtract_151a1 : Sum  Inputs=+-
  Subtract_1d9ae : Sum  Inputs=+-
  Subtract_292bb : Sum  Inputs=+-
  Subtract_6e1b4 : Sum  Inputs=+-
  Subtract_6e5ac : Sum  Inputs=+-
  Subtract_75e52 : Sum  Inputs=+-
  Subtract_b9562 : Sum  Inputs=+-
  Blockout_i_q_SG_D_2_bbd87 : Outport
  wires:
  MathFunc_sin_69210/1 -> Product_b81bd/2
  Product_6790a/1 -> Product_b81bd/1
  Constant_-1_d6b5e/1 -> Product_89ab6/1
  Constant_-1_31208/1 -> Product_5e931/1
  Constant_x_l_0134d/1 -> Product_89ab6/2
  Product_89ab6/1 -> Add_dbe16/1
  Subtract_292bb/1 -> Product_e4b88/2
  Constant_x_qdd_75035/1 -> Subtract_151a1/2
  Constant_x_qdd_c2e2f/1 -> Add_dbe16/2
  Add_d2493/1 -> Product_6790a/2
  Constant_x_l_fd7b2/1 -> Product_5e931/2
  Constant_x_qd_fd3a7/1 -> Subtract_151a1/1
  Constant_-1_df0dd/1 -> Product_ee3ef/1
  Constant_x_l_3454d/1 -> Product_ee3ef/2
  State_psi_1d_SG_D_2_3e03a/1 -> Product_8d08d/2
  State_psi_gq_SG_D_2_62065/1 -> Product_6dc77/1
  Add_dbe16/1 -> Product_6dc77/2
  Product_5e931/1 -> Add_da261/1
  Divide_62534/1 -> Add_b2275/1
  Constant_x_qd_9ab83/1 -> Add_da261/2
  State_psi_kq_SG_D_2_46994/1 -> Product_beae7/1
  Add_61347/1 -> Subtract_75e52/1
  Constant_x_ddd_709cf/1 -> Subtract_292bb/2
  Subtract_151a1/1 -> Product_beae7/2
  Product_ee3ef/1 -> Add_56e92/1
  Constant_x_qd_a957b/1 -> Add_56e92/2
  Constant_-1_d8871/1 -> Product_8d08d/1
  Constant_x_l_f5f84/1 -> Subtract_b9562/2
  Constant_x_dd_9c14e/1 -> Subtract_292bb/1
  Product_6dc77/1 -> Divide_70422/1
  Divide_d545d/1 -> Subtract_75e52/2
  Add_da261/1 -> Divide_70422/2
  Product_46ec5/1 -> Divide_36c98/1
  Product_beae7/1 -> Divide_4487d/1
  Constant_-1_31adc/1 -> Product_6790a/1
  Product_8d08d/1 -> Product_e4b88/1
  Add_56e92/1 -> Divide_4487d/2
  Constant_x_dd_b221d/1 -> Subtract_6e1b4/1
  Subtract_75e52/1 -> Product_46ec5/1
  Subtract_6e5ac/1 -> Product_7ddb9/2
  Constant_x_l_699e0/1 -> Subtract_6e1b4/2
  Constant_x_ddd_e9928/1 -> Subtract_6e5ac/1
  Constant_x_l_c5593/1 -> Subtract_6e5ac/2
  Divide_70422/1 -> Subtract_1d9ae/1
  Divide_36c98/1 -> Add_b2275/2
  Product_7ddb9/1 -> Divide_d545d/1
  Divide_4487d/1 -> Subtract_1d9ae/2
  Subtract_b9562/1 -> Divide_d545d/2
  Product_e4b88/1 -> Divide_e9059/1
  Subtract_6e1b4/1 -> Divide_e9059/2
  Constant_x_qdd_fb9fa/1 -> Divide_62534/2
  State_psi_fd_SG_D_2_212cc/1 -> Product_7ddb9/1
  Constant_x_dd_3bc88/1 -> Subtract_b9562/1
  Subtract_1d9ae/1 -> Add_d2493/1
  State_psi_q_SG_D_2_d1f7c/1 -> Add_d2493/2
  Constant_x_ddd_677e6/1 -> Divide_36c98/2
  Divide_e9059/1 -> Add_61347/1
  State_psi_d_SG_D_2_1a46c/1 -> Add_61347/2
  State_theta_SG_D_2_14f06/1 -> MathFunc_sin_69210/1
  State_theta_SG_D_2_6d11f/1 -> MathFunc_cos_56f7a/1
  MathFunc_cos_56f7a/1 -> Product_46ec5/2
  Product_b81bd/1 -> Divide_62534/1
  Add_b2275/1 -> Blockout_i_q_SG_D_2_bbd87/1

== system case2/SG_D_2/theta_SG_D_2_out_block ==
  note: theta_SG_D_2_out in case2
      | $\theta _{\mathrm{SG},D,2}$
      | Automatically generated on 2025-10-31 18:55:13 .
  State_theta_SG_D_2_6b056 : Inport
  Blockout_theta_SG_D_2_out_ba39c : Outport
  wires:
  State_theta_SG_D_2_6b056/1 -> Blockout_theta_SG_D_2_out_ba39c/1

== system case2/SG_D_2/w_SG_D_2_out_block ==
  note: w_SG_D_2_out in case2
      | $w_{\mathrm{SG},D,2}$
      | Automatically generated on 2025-10-31 18:55:12 .
  State_w_SG_D_2_b0f95 : Inport
  Blockout_w_SG_D_2_out_f6fd7 : Outport
  wires:
  State_w_SG_D_2_b0f95/1 -> Blockout_w_SG_D_2_out_f6fd7/1

== system case2/SG_D_3/T_e_SG_D_3_block ==
  note: T_e_SG_D_3 in case2
      | $-\frac{\psi _{d,\mathrm{SG},D,3}\,\left(\psi _{q,\mathrm{SG},D,3}+\frac{\psi _{\mathrm{gq},\mathrm{SG},D,3}\,\left(x_{l}-x_{\mathrm{qdd}}\right)}{x_{l}-x_{\mathrm{qd}}}+\frac{\psi _{\mathrm{kq},\mathrm{SG},D,3}\,\left(x_{\mathrm{qd}}-x_{\mathrm{qdd}}\right)}{x_{l}-x_{\mathrm{qd}}}\right)}{x_{\mathrm{qdd}}}-\frac{\psi _{q,\mathrm{SG},D,3}\,\left(\frac{\psi _{\mathrm{1d},\mathrm{SG},D,3}\,\left(x_{\mathrm{dd}}-x_{\mathrm{ddd}}\right)}{x_{\mathrm{dd}}-x_{l}}-\psi _{d,\mathrm{SG},D,3}+\frac{\psi _{\mathrm{fd},\mathrm{SG},D,3}\,\left(x_{\mathrm{ddd}}-x_{l}\right)}{x_{\mathrm{dd}}-x_{l}}\right)}{x_{\mathrm{ddd}}}$
      | Automatically generated on 2025-10-31 18:56:19 .
  State_psi_d_SG_D_3_e6750 : Inport
  State_psi_gq_SG_D_3_f5567 : Inport  Port=2
  State_psi_kq_SG_D_3_1726a : Inport  Port=3
  State_psi_q_SG_D_3_e157f : Inport  Port=4
  State_psi_q_SG_D_3_b3ce3 : Inport  Port=5
  State_psi_1d_SG_D_3_cd401 : Inport  Port=6
  State_psi_d_SG_D_3_a51a8 : Inport  Port=7
  State_psi_fd_SG_D_3_e25ec : Inport  Port=8
  Add_1b1b9 : Sum
  Add_871b7 : Sum
  Add_b7939 : Sum
  Add_bc286 : Sum
  Add_f4832 : Sum
  Add_fb2dd : Sum
  Constant_-1_6f62c : Constant  Value=-1
  Constant_-1_9ca54 : Constant  Value=-1
  Constant_-1_c2aac : Constant  Value=-1
  Constant_-1_d647e : Constant  Value=-1
  Constant_-1_e6c9a : Constant  Value=-1
  Constant_x_dd_5c89d : Constant  Value=x_dd
  Constant_x_dd_9d7de : Constant  Value=x_dd
  Constant_x_dd_f5ec9 : Constant  Value=x_dd
  Constant_x_ddd_2a172 : Constant  Value=x_ddd
  Constant_x_ddd_308bb : Constant  Value=x_ddd
  Constant_x_ddd_b5c8a : Constant  Value=x_ddd
  Constant_x_l_25361 : Constant  Value=x_l
  Constant_x_l_364f5 : Constant  Value=x_l
  Constant_x_l_4e011 : Constant  Value=x_l
  Constant_x_l_bc462 : Constant  Value=x_l
  Constant_x_l_d4d4d : Constant  Value=x_l
  Constant_x_l_e594e : Constant  Value=x_l
  Constant_x_qd_85d7b : Constant  Value=x_qd
  Constant_x_qd_c6bd1 : Constant  Value=x_qd
  Constant_x_qd_e7e6b : Constant  Value=x_qd
  Constant_x_qdd_3555f : Constant  Value=x_qdd
  Constant_x_qdd_4e53c : Constant  Value=x_qdd
  Constant_x_qdd_6496b : Constant  Value=x_qdd
  Divide_325a2 : Product  Inputs=*/
  Divide_4cffd : Product  Inputs=*/
  Divide_79d80 : Product  Inputs=*/
  Divide_8be83 : Product  Inputs=*/
  Divide_9f55b : Product  Inputs=*/
  Divide_a4440 : Product  Inputs=*/
  Product_1b474 : Product
  Product_288b6 : Product
  Product_3f33f : Product
  Product_4033a : Product
  Product_6fe81 : Product
  Product_a81ff : Product
  Product_aeae6 : Product
  Product_b5e31 : Product
  Product_c198a : Product
  Product_df941 : Product
  Product_ed3ac : Product
  Subtract_111b1 : Sum  Inputs=+-
  Subtract_a87d3 : Sum  Inputs=+-
  Subtract_ac372 : Sum  Inputs=+-
  Subtract_c33bf : Sum  Inputs=+-
  Subtract_cc2b4 : Sum  Inputs=+-
  Subtract_d761a : Sum  Inputs=+-
  Subtract_d8cee : Sum  Inputs=+-
  Blockout_T_e_SG_D_3_6da4d : Outport
  wires:
  State_psi_q_SG_D_3_e157f/1 -> Add_fb2dd/2
  Constant_-1_e6c9a/1 -> Product_ed3ac/1
  Subtract_cc2b4/1 -> Product_4033a/2
  State_psi_1d_SG_D_3_cd401/1 -> Product_3f33f/2
  Constant_-1_6f62c/1 -> Product_df941/1
  Constant_x_l_25361/1 -> Product_df941/2
  Add_bc286/1 -> Subtract_cc2b4/1
  State_psi_d_SG_D_3_a51a8/1 -> Add_bc286/2
  Product_df941/1 -> Add_871b7/1
  Constant_x_qdd_6496b/1 -> Subtract_c33bf/2
  Add_fb2dd/1 -> Product_b5e31/2
  Constant_x_qdd_3555f/1 -> Add_871b7/2
  State_psi_q_SG_D_3_b3ce3/1 -> Product_4033a/1
  Constant_x_l_d4d4d/1 -> Product_ed3ac/2
  Subtract_a87d3/1 -> Divide_4cffd/2
  Constant_x_l_4e011/1 -> Subtract_111b1/2
  Constant_x_qd_e7e6b/1 -> Subtract_c33bf/1
  Constant_-1_9ca54/1 -> Product_aeae6/1
  Subtract_d8cee/1 -> Divide_9f55b/2
  Constant_x_l_364f5/1 -> Product_aeae6/2
  Product_a81ff/1 -> Divide_9f55b/1
  Constant_-1_c2aac/1 -> Product_3f33f/1
  Product_3f33f/1 -> Product_a81ff/1
  Constant_x_dd_9d7de/1 -> Subtract_d761a/1
  Constant_x_ddd_2a172/1 -> Subtract_d761a/2
  Add_f4832/1 -> Blockout_T_e_SG_D_3_6da4d/1
  State_psi_gq_SG_D_3_f5567/1 -> Product_c198a/1
  Product_4033a/1 -> Divide_79d80/1
  Add_871b7/1 -> Product_c198a/2
  State_psi_fd_SG_D_3_e25ec/1 -> Product_1b474/1
  Product_ed3ac/1 -> Add_1b1b9/1
  Constant_x_qd_85d7b/1 -> Add_1b1b9/2
  Constant_x_dd_f5ec9/1 -> Subtract_d8cee/1
  State_psi_kq_SG_D_3_1726a/1 -> Product_288b6/1
  Constant_x_dd_5c89d/1 -> Subtract_a87d3/1
  Subtract_c33bf/1 -> Product_288b6/2
  Product_b5e31/1 -> Divide_325a2/1
  Product_aeae6/1 -> Add_b7939/1
  Add_1b1b9/1 -> Divide_8be83/2
  Constant_x_qd_c6bd1/1 -> Add_b7939/2
  Subtract_d761a/1 -> Product_a81ff/2
  Constant_x_l_e594e/1 -> Subtract_d8cee/2
  Constant_x_ddd_b5c8a/1 -> Subtract_111b1/1
  Product_c198a/1 -> Divide_8be83/1
  Product_288b6/1 -> Divide_a4440/1
  Add_b7939/1 -> Divide_a4440/2
  Constant_x_ddd_308bb/1 -> Divide_79d80/2
  Subtract_111b1/1 -> Product_1b474/2
  Divide_8be83/1 -> Subtract_ac372/1
  Constant_x_l_bc462/1 -> Subtract_a87d3/2
  Divide_a4440/1 -> Subtract_ac372/2
  Divide_9f55b/1 -> Add_bc286/1
  Product_1b474/1 -> Divide_4cffd/1
  Constant_-1_d647e/1 -> Product_6fe81/1
  State_psi_d_SG_D_3_e6750/1 -> Product_6fe81/2
  Subtract_ac372/1 -> Add_fb2dd/1
  Divide_4cffd/1 -> Subtract_cc2b4/2
  Product_6fe81/1 -> Product_b5e31/1
  Constant_x_qdd_4e53c/1 -> Divide_325a2/2
  Divide_325a2/1 -> Add_f4832/1
  Divide_79d80/1 -> Add_f4832/2

== system case2/SG_D_3/d_E_fd_SG_D_3_block ==
  note: d_E_fd_SG_D_3 in case2
      | $\frac{V_{f,\mathrm{SG},D,3}-E_{\mathrm{fd},\mathrm{SG},D,3}\,K_{E}}{T_{E}}$
      | Automatically generated on 2025-10-31 18:56:04 .
  State_E_fd_SG_D_3_97dd1 : Inport
  State_V_f_SG_D_3_e8d17 : Inport  Port=2
  Add_f82c8 : Sum
  Constant_-1_f4527 : Constant  Value=-1
  Constant_K_E_e2377 : Constant  Value=K_E
  Constant_T_E_00078 : Constant  Value=T_E
  Divide_666a3 : Product  Inputs=*/
  Product_18dec : Product
  Product_bb221 : Product
  Blockout_d_E_fd_SG_D_3_4d917 : Outport
  wires:
  State_V_f_SG_D_3_e8d17/1 -> Add_f82c8/2
  Constant_-1_f4527/1 -> Product_18dec/1
  State_E_fd_SG_D_3_97dd1/1 -> Product_18dec/2
  Constant_T_E_00078/1 -> Divide_666a3/2
  Product_18dec/1 -> Product_bb221/1
  Product_bb221/1 -> Add_f82c8/1
  Constant_K_E_e2377/1 -> Product_bb221/2
  Divide_666a3/1 -> Blockout_d_E_fd_SG_D_3_4d917/1
  Add_f82c8/1 -> Divide_666a3/1

== system case2/SG_D_3/d_Px_1_SG_D_3_block ==
  note: d_Px_1_SG_D_3 in case2
      | $\frac{w_{\mathrm{SG},D,3}-2\,\pi \,f_{0}}{T_{w}}-\frac{\mathrm{Px}_{1,\mathrm{SG},D,3}}{T_{w}}$
      | Automatically generated on 2025-10-31 18:56:05 .
  State_Px_1_SG_D_3_6a762 : Inport
  State_w_SG_D_3_fb455 : Inport  Port=2
  Add_05e36 : Sum
  Add_923ad : Sum
  Constant_-1_b9606 : Constant  Value=-1
  Constant_-2.0_c2d29 : Constant  Value=-2.0
  Constant_T_w_15b3e : Constant  Value=T_w
  Constant_T_w_50d4c : Constant  Value=T_w
  Constant_f0_a0a63 : Constant  Value=f0
  Constant_pi_258b0 : Constant  Value=pi
  Divide_091fb : Product  Inputs=*/
  Divide_f8577 : Product  Inputs=*/
  Product_6162c : Product
  Product_63fc4 : Product
  Product_b2b18 : Product
  Blockout_d_Px_1_SG_D_3_ecaac : Outport
  wires:
  Constant_f0_a0a63/1 -> Product_63fc4/2
  Constant_-1_b9606/1 -> Product_6162c/1
  Constant_-2.0_c2d29/1 -> Product_b2b18/1
  Constant_pi_258b0/1 -> Product_b2b18/2
  Product_b2b18/1 -> Product_63fc4/1
  State_w_SG_D_3_fb455/1 -> Add_05e36/2
  Divide_f8577/1 -> Add_923ad/1
  State_Px_1_SG_D_3_6a762/1 -> Product_6162c/2
  Product_63fc4/1 -> Add_05e36/1
  Product_6162c/1 -> Divide_f8577/1
  Constant_T_w_15b3e/1 -> Divide_f8577/2
  Add_05e36/1 -> Divide_091fb/1
  Constant_T_w_50d4c/1 -> Divide_091fb/2
  Divide_091fb/1 -> Add_923ad/2
  Add_923ad/1 -> Blockout_d_Px_1_SG_D_3_ecaac/1

== system case2/SG_D_3/d_Px_2_SG_D_3_block ==
  note: d_Px_2_SG_D_3 in case2
      | $\frac{\mathrm{Px}_{1,\mathrm{SG},D,3}-T_{2}\,\left(\frac{\mathrm{Px}_{1,\mathrm{SG},D,3}}{T_{w}}-\frac{w_{\mathrm{SG},D,3}-2\,\pi \,f_{0}}{T_{w}}\right)}{T_{1}}-\frac{\mathrm{Px}_{2,\mathrm{SG},D,3}}{T_{1}}$
      | Automatically generated on 2025-10-31 18:56:07 .
  State_Px_2_SG_D_3_e4ce9 : Inport
  State_Px_1_SG_D_3_07a77 : Inport  Port=2
  State_Px_1_SG_D_3_de3ab : Inport  Port=3
  State_w_SG_D_3_9f660 : Inport  Port=4
  Add_0bbff : Sum
  Add_61389 : Sum
  Add_d96b1 : Sum
  Add_e8c06 : Sum
  Constant_-1_0b61e : Constant  Value=-1
  Constant_-1_21d80 : Constant  Value=-1
  Constant_-2.0_00679 : Constant  Value=-2.0
  Constant_T_1_2a755 : Constant  Value=T_1
  Constant_T_1_2b6f9 : Constant  Value=T_1
  Constant_T_2_3bc05 : Constant  Value=T_2
  Constant_T_w_24db9 : Constant  Value=T_w
  Constant_T_w_eb6b0 : Constant  Value=T_w
  Constant_f0_dfd19 : Constant  Value=f0
  Constant_pi_c4ff2 : Constant  Value=pi
  Divide_0c73e : Product  Inputs=*/
  Divide_1ef8d : Product  Inputs=*/
  Divide_26253 : Product  Inputs=*/
  Divide_927e2 : Product  Inputs=*/
  Product_552b6 : Product
  Product_5ea71 : Product
  Product_afcf8 : Product
  Product_dcada : Product
  Product_f83ad : Product
  Blockout_d_Px_2_SG_D_3_b7721 : Outport
  wires:
  State_Px_1_SG_D_3_de3ab/1 -> Product_dcada/2
  Constant_-2.0_00679/1 -> Product_552b6/1
  Constant_f0_dfd19/1 -> Product_5ea71/2
  Constant_pi_c4ff2/1 -> Product_552b6/2
  Product_552b6/1 -> Product_5ea71/1
  State_w_SG_D_3_9f660/1 -> Add_e8c06/2
  Constant_-1_0b61e/1 -> Product_dcada/1
  Product_5ea71/1 -> Add_e8c06/1
  Product_dcada/1 -> Divide_26253/1
  Constant_T_w_24db9/1 -> Divide_26253/2
  Add_e8c06/1 -> Divide_1ef8d/1
  Constant_T_w_eb6b0/1 -> Divide_1ef8d/2
  Divide_26253/1 -> Add_61389/1
  Divide_1ef8d/1 -> Add_61389/2
  Constant_T_2_3bc05/1 -> Product_afcf8/1
  Add_61389/1 -> Product_afcf8/2
  Constant_-1_21d80/1 -> Product_f83ad/1
  Product_afcf8/1 -> Add_0bbff/2
  State_Px_2_SG_D_3_e4ce9/1 -> Product_f83ad/2
  State_Px_1_SG_D_3_07a77/1 -> Add_0bbff/1
  Product_f83ad/1 -> Divide_0c73e/1
  Add_d96b1/1 -> Blockout_d_Px_2_SG_D_3_b7721/1
  Constant_T_1_2b6f9/1 -> Divide_0c73e/2
  Add_0bbff/1 -> Divide_927e2/1
  Constant_T_1_2a755/1 -> Divide_927e2/2
  Divide_0c73e/1 -> Add_d96b1/1
  Divide_927e2/1 -> Add_d96b1/2

== system case2/SG_D_3/d_Px_3_SG_D_3_block ==
  note: d_Px_3_SG_D_3 in case2
      | $\frac{\mathrm{Px}_{2,\mathrm{SG},D,3}+T_{4}\,\left(\frac{\mathrm{Px}_{1,\mathrm{SG},D,3}-T_{2}\,\left(\frac{\mathrm{Px}_{1,\mathrm{SG},D,3}}{T_{w}}-\frac{w_{\mathrm{SG},D,3}-2\,\pi \,f_{0}}{T_{w}}\right)}{T_{1}}-\frac{\mathrm{Px}_{2,\mathrm{SG},D,3}}{T_{1}}\right)}{T_{3}}-\frac{\mathrm{Px}_{3,\mathrm{SG},D,3}}{T_{3}}$
      | Automatically generated on 2025-10-31 18:56:10 .
  State_Px_3_SG_D_3_99451 : Inport
  State_Px_2_SG_D_3_6ab48 : Inport  Port=2
  State_Px_2_SG_D_3_b9577 : Inport  Port=3
  State_Px_1_SG_D_3_dfdda : Inport  Port=4
  State_Px_1_SG_D_3_46ef9 : Inport  Port=5
  State_w_SG_D_3_a9ec3 : Inport  Port=6
  Add_3ccb5 : Sum
  Add_3f121 : Sum
  Add_42b6c : Sum
  Add_673ab : Sum
  Add_8f3f9 : Sum
  Add_bdda4 : Sum
  Constant_-1_16f45 : Constant  Value=-1
  Constant_-1_8020b : Constant  Value=-1
  Constant_-1_db2f3 : Constant  Value=-1
  Constant_-2.0_e180f : Constant  Value=-2.0
  Constant_T_1_74870 : Constant  Value=T_1
  Constant_T_1_96281 : Constant  Value=T_1
  Constant_T_2_76cc4 : Constant  Value=T_2
  Constant_T_3_5f8ef : Constant  Value=T_3
  Constant_T_3_87f58 : Constant  Value=T_3
  Constant_T_4_9b431 : Constant  Value=T_4
  Constant_T_w_61770 : Constant  Value=T_w
  Constant_T_w_c4d3b : Constant  Value=T_w
  Constant_f0_ef753 : Constant  Value=f0
  Constant_pi_e3ed9 : Constant  Value=pi
  Divide_218dc : Product  Inputs=*/
  Divide_76e0f : Product  Inputs=*/
  Divide_81b69 : Product  Inputs=*/
  Divide_9c7fc : Product  Inputs=*/
  Divide_c2b24 : Product  Inputs=*/
  Divide_c8e50 : Product  Inputs=*/
  Product_10482 : Product
  Product_2dfa3 : Product
  Product_356b9 : Product
  Product_a8740 : Product
  Product_d60c1 : Product
  Product_d8dda : Product
  Product_d8e4b : Product
  Blockout_d_Px_3_SG_D_3_317cb : Outport
  wires:
  State_Px_1_SG_D_3_46ef9/1 -> Product_d8e4b/2
  Constant_f0_ef753/1 -> Product_d60c1/2
  Constant_-2.0_e180f/1 -> Product_2dfa3/1
  Add_42b6c/1 -> Divide_9c7fc/1
  Constant_pi_e3ed9/1 -> Product_2dfa3/2
  Product_2dfa3/1 -> Product_d60c1/1
  State_w_SG_D_3_a9ec3/1 -> Add_3f121/2
  Constant_T_w_61770/1 -> Divide_76e0f/2
  Constant_-1_8020b/1 -> Product_d8e4b/1
  Product_d60c1/1 -> Add_3f121/1
  Product_d8e4b/1 -> Divide_76e0f/1
  Add_3f121/1 -> Divide_218dc/1
  Product_10482/1 -> Divide_81b69/1
  Constant_T_w_c4d3b/1 -> Divide_218dc/2
  Divide_76e0f/1 -> Add_bdda4/1
  Divide_218dc/1 -> Add_bdda4/2
  Constant_T_2_76cc4/1 -> Product_356b9/1
  Add_bdda4/1 -> Product_356b9/2
  Constant_-1_db2f3/1 -> Product_10482/1
  State_Px_2_SG_D_3_b9577/1 -> Product_10482/2
  State_Px_1_SG_D_3_dfdda/1 -> Add_42b6c/1
  Constant_T_3_5f8ef/1 -> Divide_c8e50/2
  Product_356b9/1 -> Add_42b6c/2
  Constant_T_1_74870/1 -> Divide_81b69/2
  Add_3ccb5/1 -> Product_d8dda/2
  Constant_T_1_96281/1 -> Divide_9c7fc/2
  Divide_c2b24/1 -> Add_8f3f9/2
  Divide_81b69/1 -> Add_3ccb5/1
  Divide_9c7fc/1 -> Add_3ccb5/2
  Constant_T_4_9b431/1 -> Product_d8dda/1
  Constant_-1_16f45/1 -> Product_a8740/1
  State_Px_3_SG_D_3_99451/1 -> Product_a8740/2
  State_Px_2_SG_D_3_6ab48/1 -> Add_673ab/1
  Product_d8dda/1 -> Add_673ab/2
  Product_a8740/1 -> Divide_c8e50/1
  Add_673ab/1 -> Divide_c2b24/1
  Constant_T_3_87f58/1 -> Divide_c2b24/2
  Divide_c8e50/1 -> Add_8f3f9/1
  Add_8f3f9/1 -> Blockout_d_Px_3_SG_D_3_317cb/1
